simulink model "Model_Simscape"  (R2023a)
settings: Solver=VariableStepAuto  StartTime=0.0  StopTime=10.0  RelTol=1e-3
model workspace (MAT data in the model file):
  Air_density = 1.29
  Body_Temperature = 37
  CtrlData_Max = 100
  CtrlData_Min = 0
  Detpress_to_Vavle : object (value not decoded)
  E_respriatory = 10
  ExpValve : object (value not decoded)
  FRC = 2
  Fan : object (value not decoded)
  FanHousing : object (value not decoded)
  Flow_Resistance_1 : object (value not decoded)
  Flow_Resistance_2 : object (value not decoded)
  Hard_Stop : Lower_bound (value not decoded)
  InspValve : object (value not decoded)
  L_to_m3 = 0.001
  Mask : object (value not decoded)
  OxyValve : object (value not decoded)
  OxygenSensor : object (value not decoded)
  Pa_to_cmH2O = 0.0101974428892
  Percent_to_Unit = 0.01
  Pipe_1 : object (value not decoded)
  Pipe_2 : object (value not decoded)
  Pipe_3 : object (value not decoded)
  R_respiratory = 2
  Reservoir : Cross_area (value not decoded)
  Trachea : object (value not decoded)
  Volume_Max = 0.9
  cmH2O_to_Pa = 98.0638
  cmH2O_to_kPa = 0.0981
  lung : object (value not decoded)
  percentage_to_rpm = 600
symbols that are objects in the model workspace (value not decoded): ExpValve, FanHousing, Flow_Resistance_1, Flow_Resistance_2, InspValve, lung, OxygenSensor
libraries: fl_lib x81, nesl_utility x17, SimscapeFluids_lib x4, aerolibatmos2 x1
(part 2 of 4)

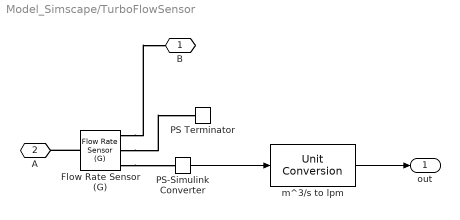
== system Model_Simscape/TurboFlowSensor ==
  Flow Rate Sensor (G) : fl_lib/Gas/Sensors/Flow Rate Sensor (G)  mass_flow_measure=true  volumetric_flow_measure=true  volumetric_flow_conditions=foundation.enum.volumetric_flow_conditions.actual  p_std=0.101325 MPa  T_std=20 degC  energy_flow_measure=false
      settings: InternalSimscapePortConfiguration="{\"Bottom\":[],\"Left\":[{\"id\":\"A\",\"label\":\"A\",\"type\":\"foundation.gas.gas\"}],\"Right\":[{\"id\":\"B\",\"label\":\"B\",\"type\":\"foundation.gas.gas\"},{\"id\":\"M\",\"label\":\"M\",\"type\":\"output\"},{\"id\":\"V\",\"label\":\"V\",\"type\":\"output\"}],\"Top\":[]}"
  PS Terminator : fl_lib/Physical Signals/Sinks/PS Terminator
  PS-Simulink Converter : nesl_utility/PS-Simulink Converter  PhysicalDomain=network_engine_domain  SubClassName=ps_output  LeftPortType=input  RightPortType=output  PseudoPeriodic=off  Frequencies=[]  VectorFormat=inherit  Unit=m^3/s  AffineConversion=off
  m^3/s to lpm : UnitConversion
  B : PMIOPort  Side=Right
  A : PMIOPort  Port=2  Side=Left
  out : Outport  Unit=lpm
  wires:
  m^3/s to lpm/1 -> out/1
  PS-Simulink Converter/1 -> m^3/s to lpm/1
  connections:
  Flow Rate Sensor (G)/RConn3 -- PS-Simulink Converter/LConn1
  Flow Rate Sensor (G)/RConn2 -- PS Terminator/LConn1
  Flow Rate Sensor (G)/LConn1 -- A/RConn1
  Flow Rate Sensor (G)/RConn1 -- B/RConn1
